simulink model "voltagemonitor"  (R2018b)
settings: Solver=VariableStepAuto  StartTime=0.0  StopTime=10.0  RelTol=1e-3
libraries: simulink x2
settings Model: Creator=diktux  LastModifiedBy=diktux

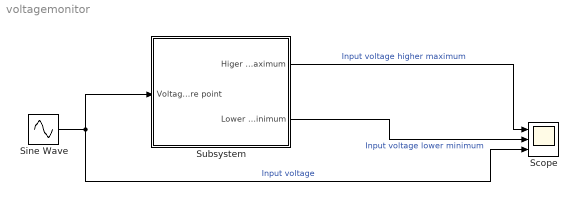
== system voltagemonitor ==
  Scope : Scope  NumInputPorts=3
  Sine Wave : Sin  Amplitude=1.5  Bias=3.5  SampleTime=0
  Subsystem : Subsystem
  wires:
  Sine Wave/1 -> Subsystem/1(Voltage measure point), Scope/3  "Input voltage"
  Subsystem/1(Higer then maximum) -> Scope/1  "Input voltage higher maximum"
  Subsystem/2(Lower then minimum) -> Scope/2  "Input voltage lower minimum"

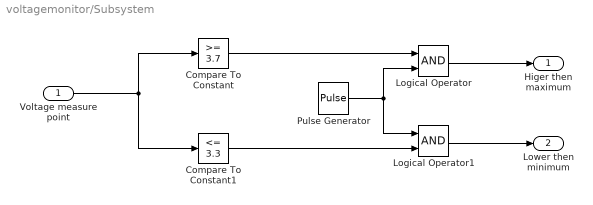
== system voltagemonitor/Subsystem ==
  Voltage measure point : Inport
  Compare To Constant : simulink/Logic and Bit Operations/Compare To Constant  relop=>=  const=3.7  OutDataTypeStr=boolean
  Compare To Constant1 : simulink/Logic and Bit Operations/Compare To Constant  relop=<=  const=3.3  OutDataTypeStr=boolean
  Logical Operator : Logic  AllPortsSameDT=off  OutDataTypeStr=boolean
  Logical Operator1 : Logic  AllPortsSameDT=off  OutDataTypeStr=boolean
  Pulse Generator : DiscretePulseGenerator  PulseType=Time based  Period=1  PulseWidth=50
  Higer then maximum : Outport
  Lower then minimum : Outport  Port=2
  wires:
  Compare To Constant1/1 -> Logical Operator1/2
  Pulse Generator/1 -> Logical Operator1/1, Logical Operator/2
  Logical Operator1/1 -> Lower then minimum/1
  Voltage measure point/1 -> Compare To Constant/1, Compare To Constant1/1
  Logical Operator/1 -> Higer then maximum/1
  Compare To Constant/1 -> Logical Operator/1
